simulink library "m_3SPS"  (R2017a)
settings: Solver=VariableStepAuto  StartTime=0.0  StopTime=10.0  RelTol=1e-3
libraries: mblibv1 x31
settings Model: Creator=ivanp7  LastModifiedBy=ivanp7

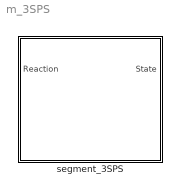
== system m_3SPS ==
  segment_3SPS : Subsystem  mask{segment_turn=0, platform_mass=0, platform_width=0, platform_thickness=0, platform_inertia=[0 0 0; 0 0 0; 0 0 0], mechanism_mass=0, mechanism_height=0, base_width=0, piston_mass=0, piston_inertia=[0 0 0; 0 0 0; 0 0 0], cylinder_inertia=[0 0 0; 0 0 0; 0 0 0]}
      mask prompts: segment_turn "Segment turn angle"; platform_mass "Platform mass, kg"; platform_width "Platform width, m"; platform_thickness "Platform thickness, m"; platform_inertia "Platform momentum of inertia matrix, kg*m^2"; mechanism_mass "Mechanism mass, kg"; mechanism_height "Mechanism height, m"; base_width "Base width, m"; piston_mass ""Piston" mass"; piston_inertia ""Piston" momentum of inertia matrix, kg*m^2"; cylinder_inertia ""Cylinder" momentum of inertia matrix, kg*m^2"
      mask init:
      | platform_radius = platform_width/2;
      | base_radius = base_width/2;
      | p_length = sqrt(mechanism_height^2 + (base_radius-platform_radius)^2);
      | 
      | q0 = [([1 1 1] * sign(base_radius-platform_radius) * sqrt((1 - mechanism_height / sqrt(mechanism_height^2 + (base_radius-platform_radius)^2)) / 2))  sqrt((1 + mechanism_height / sqrt(mechanism_height^2 + (base_radius-platform_radius)^2)) / 2)];
      | p1_quaternion = [[1 0 0] 1] .* q0;
      | p2_quaternion = [[-1/2 -sqrt(3)/2 0] 1] .* q0;
      | p3_quaternion = [[-1/2 sqrt(3)/2 0] 1] .* q0;
      | 
      | cylinder_mass = mechanism_mass/3 - piston_mass;
      mask DialogControl Container_plat_param Prompt: Platform parameters
      mask DialogControl Container_mech_param Prompt: Mechanism parameters
      mask DialogControl Container_mech_add_param Prompt: Additional mechanism parameters

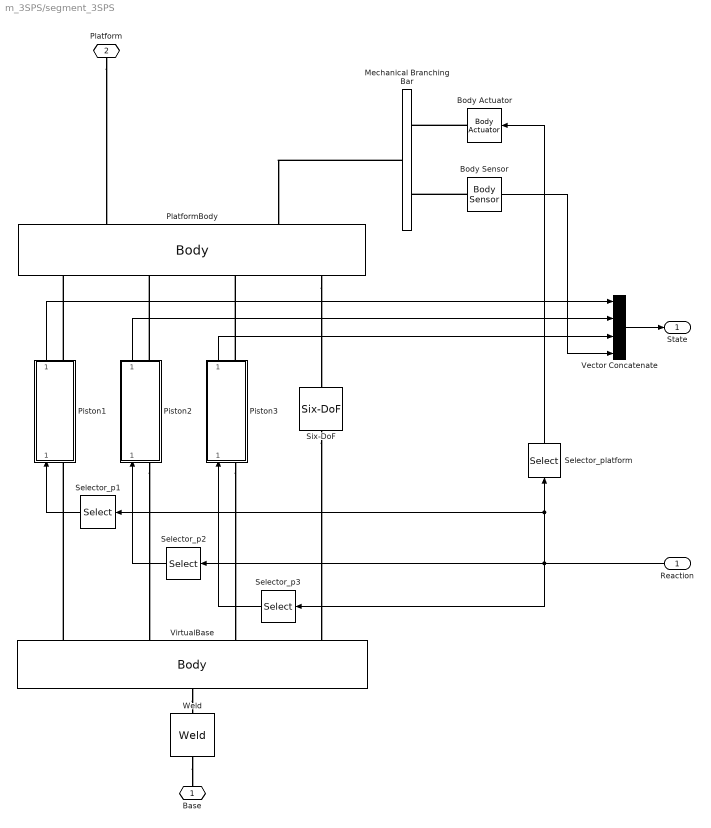
== system m_3SPS/segment_3SPS ==
  Reaction : Inport  OutDataTypeStr=double
  Body Actuator : mblibv1/Sensors &  Actuators/Body Actuator  UpdateFromCAD=off  PhysicalDomain=Mechanical  PortType=blob  ActuationStyle=Force  AngleUnits=deg  ArcVelocityUnits=deg/s  ArcAccelerationUnits=deg/s^2  CoordPositionUnits=m  VelocityUnits=m/s  AccelerationUnits=m/s^2  ForceUnits=N  TorqueUnits=N*m  ActiveIO=off  Width=1  DialogClass=MechanicalActuatorBlock  ReferenceFrame=Absolute (World)  Angle=off  CoordPosition=on  Force=on  Torque=on
      settings: SourceProductName=Simscape Multibody  SourceProductBaseCode=MS
  Body Sensor : mblibv1/Sensors &  Actuators/Body Sensor  UpdateFromCAD=off  PhysicalDomain=Mechanical  PortType=blob  Muxed=on  Pose=on  Angle=on  AngleUnits=deg  ArcVelocity=on  ArcVelocityUnits=rad/s  ArcAcceleration=on  ArcAccelerationUnits=rad/s^2  CoordPosition=on  CoordPositionUnits=m  Velocity=on  VelocityUnits=m/s  Acceleration=on  AccelerationUnits=m/s^2  Quaternion=on  QuaternionDT=off  QuaternionDDT=off  QuaternionUnits=off  OutputVector=[1]  ActiveIO=off  Width=1  DialogClass=MechanicalSensorBlock  ReferenceFrame=Absolute (World)
      settings: SourceProductName=Simscape Multibody  SourceProductBaseCode=MS
  Mechanical Branching Bar : mblibv1/Utilities/Mechanical Branching Bar  LConnTagsString=_newl0  RConnTagsString=SA0|SA1  UpdateFromCAD=off  DialogClass=MechanicalBranchingBarBlock  NumSAPorts=2
      settings: SourceProductName=Simscape Multibody  SourceProductBaseCode=MS
  Piston1 : Subsystem
  Piston2 : Subsystem
  Piston3 : Subsystem
  PlatformBody : mblibv1/Bodies/Body  LConnTagsString=CS5|CS6  RConnTagsString=CS1|CS2|CS3|CS4  UpdateFromCAD=off  DialogClass=MechanicalBodyBlock  Mass=platform_mass  MassUnits=kg  InertiaUnits=kg*m^2  Inertia=platform_inertia  Shape=Cylinder  ShapeDims=[1 1]  ShapeUnits=m  ShapeUse=false  Density=1  DensityUnits=kg/m^3  DensityUse=false  GraphicsMode=EQELLIPSE  BodyColorSelMode=MACHINE_DEFAULT  BodyColor=[1 0 0]  AttachedToCS=CG  CG=Left$CG$[0 0 platform_thickness/2]$CS4$CS4$m$[0 0 0]$Euler X-Y-Z$deg$CS4$false$none  WorkingFrames=Right$CS1$[0 0 0]$Adjoining$Adjoining$m$[0 0 0]$Euler X-Y-Z$deg$CS4$true$none#Right$CS2$[0 0 0]$Adjoining$Adjoining$m$[0 0 0]$Euler X-Y-Z$deg$CS4$true$none#Right$CS3$[0 0 0]$Adjoining$Adjoining$m$[0 0 0]$Euler X-Y-Z$deg$CS4$true$none#Right$CS4$[0 0 mechanism_height]$Adjoining$Adjoining$m$[0 0 0]$Euler X-Y-Z$deg$Adjoining$true$none#Left$CS5$[0 0 platform_thickness]$CS4$CS4$m$[0 0 0]$Euler X-Y-Z$deg$CS4$true$none#Left$CS6$[0 0 0]$CS5$CS5$m$[0 0 0]$Euler X-Y-Z$deg$CG$true$none  CGPos=[0 0 platform_thickness/2]  CGRot=[0 0 0]  CS0Pos=[]  CS0Rot=[]  CS1Pos=[0 0 0]  CS1Rot=[0 0 0]  CS2Pos=[0 0 0]  CS2Rot=[0 0 0]  CS3Pos=[0 0 0]  CS3Rot=[0 0 0]  CS4Pos=[0 0 mechanism_height]  CS4Rot=[0 0 0]  CS5Pos=[0 0 platform_thickness]  CS5Rot=[0 0 0]  CS6Pos=[0 0 0]  CS6Rot=[0 0 0]  CS7Pos=[]  CS7Rot=[]  CS8Pos=[]  CS8Rot=[]  CS9Pos=[]  CS9Rot=[]  CS10Pos=[]  CS10Rot=[]  CS11Pos=[]  CS11Rot=[]  CS12Pos=[]  CS12Rot=[]  CS13Pos=[]  CS13Rot=[]  CS14Pos=[]  CS14Rot=[]  CS15Pos=[]  CS15Rot=[]  CS16Pos=[]  CS16Rot=[]  CS17Pos=[]  CS17Rot=[]  CS18Pos=[]  CS18Rot=[]  CS19Pos=[]  CS19Rot=[]  CS20Pos=[]  CS20Rot=[]
      settings: SourceProductName=Simscape Multibody  SourceProductBaseCode=MS
  Selector_p1 : Selector  InputPortWidth=9  IndexOptions=Index vector (dialog)  Indices=[1]  OutputSizes=1
  Selector_p2 : Selector  InputPortWidth=9  IndexOptions=Index vector (dialog)  Indices=[2]  OutputSizes=1
  Selector_p3 : Selector  InputPortWidth=9  IndexOptions=Index vector (dialog)  Indices=[3]  OutputSizes=1
  Selector_platform : Selector  InputPortWidth=9  IndexOptions=Index vector (dialog)  Indices=[4 5 6 7 8 9]  OutputSizes=1
  Six-DoF : mblibv1/Joints/Six-DoF  LConnTagsString=__newl0  RConnTagsString=__newr0  UpdateFromCAD=off  NumSAPorts=0  CutJoint=off  MarkAsCut=off  Primitives=prismatic_prismatic  PrimitiveProps=P1$WORLD$[1 0 0]$prismatic#P2$WORLD$[0 1 0]$prismatic#P3$WORLD$[0 0 1]$prismatic#S$WORLD$[0 0 0]$spherical  DialogClass=JointBlock  P1Axis=[1 0 0]  P2Axis=[0 1 0]  P3Axis=[0 0 1]  SAxis=[0 0 0]
      settings: SourceProductName=Simscape Multibody  SourceProductBaseCode=MS
  Vector Concatenate : Concatenate  NumInputs=4
  VirtualBase : mblibv1/Bodies/Body  LConnTagsString=CS1|CS2|CS3|CS4  RConnTagsString=CG  UpdateFromCAD=off  DialogClass=MechanicalBodyBlock  Mass=0  MassUnits=kg  InertiaUnits=kg*m^2  Inertia=zeros(3)  Shape=Cylinder  ShapeDims=[1 1]  ShapeUnits=m  ShapeUse=false  Density=1  DensityUnits=kg/m^3  DensityUse=false  GraphicsMode=EQELLIPSE  BodyColorSelMode=MACHINE_DEFAULT  BodyColor=[1 0 0]  AttachedToCS=CG  CG=Right$CG$[0 0 0]$Adjoining$Adjoining$m$[0 0 segment_turn]$Euler X-Y-Z$deg$Adjoining$true$none  WorkingFrames=Left$CS1$[0 base_radius 0]$CG$CG$m$[0 0 0]$Euler X-Y-Z$deg$CG$true$none#Left$CS2$[sqrt(3)*base_radius/2 -base_radius/2 0]$CG$CG$m$[0 0 0]$Euler X-Y-Z$deg$CG$true$none#Left$CS3$[-sqrt(3)*base_radius/2 -base_radius/2 0]$CG$CG$m$[0 0 0]$Euler X-Y-Z$deg$CG$true$none#Left$CS4$[0 0 0]$CG$CG$m$[0 0 0]$Euler X-Y-Z$deg$CG$true$none  CGPos=[0 0 0]  CGRot=[0 0 segment_turn]  CS0Pos=[]  CS0Rot=[]  CS1Pos=[0 base_radius 0]  CS1Rot=[0 0 0]  CS2Pos=[sqrt(3)*base_radius/2 -base_radius/2 0]  CS2Rot=[0 0 0]  CS3Pos=[-sqrt(3)*base_radius/2 -base_radius/2 0]  CS3Rot=[0 0 0]  CS4Pos=[0 0 0]  CS4Rot=[0 0 0]  CS5Pos=[]  CS5Rot=[]  CS6Pos=[]  CS6Rot=[]  CS7Pos=[]  CS7Rot=[]  CS8Pos=[]  CS8Rot=[]  CS9Pos=[]  CS9Rot=[]  CS10Pos=[]  CS10Rot=[]  CS11Pos=[]  CS11Rot=[]  CS12Pos=[]  CS12Rot=[]  CS13Pos=[]  CS13Rot=[]  CS14Pos=[]  CS14Rot=[]  CS15Pos=[]  CS15Rot=[]  CS16Pos=[]  CS16Rot=[]  CS17Pos=[]  CS17Rot=[]  CS18Pos=[]  CS18Rot=[]  CS19Pos=[]  CS19Rot=[]  CS20Pos=[]  CS20Rot=[]
      settings: SourceProductName=Simscape Multibody  SourceProductBaseCode=MS
  Weld : mblibv1/Joints/Weld  LConnTagsString=__newl0  RConnTagsString=__newr0  UpdateFromCAD=off  NumSAPorts=0  CutJoint=off  MarkAsCut=off  Primitives=weld  PrimitiveProps=W$WORLD$[0 0 0]$weld  DialogClass=JointBlock  WAxis=[0 0 0]
      settings: SourceProductName=Simscape Multibody  SourceProductBaseCode=MS
  Base : PMIOPort  Port=1  Side=Left
  Platform : PMIOPort  Port=2  Side=Right
  State : Outport  OutDataTypeStr=double
  wires:
  Piston1/1(P1_State) -> Vector Concatenate/1
  Piston2/1(P2_State) -> Vector Concatenate/2
  Piston3/1(P3_State) -> Vector Concatenate/3
  Reaction/1 -> Selector_p3/1, Selector_p1/1, Selector_platform/1, Selector_p2/1
  Vector Concatenate/1 -> State/1
  Body Sensor/1 -> Vector Concatenate/4
  Selector_platform/1 -> Body Actuator/1
  Selector_p1/1 -> Piston1/1(P1_Reaction)
  Selector_p2/1 -> Piston2/1(P2_Reaction)
  Selector_p3/1 -> Piston3/1(P3_Reaction)
  connections:
  Weld/LConn1 -- Base/RConn1
  VirtualBase/RConn1 -- Weld/RConn1
  Piston1/RConn1 -- PlatformBody/RConn1
  VirtualBase/LConn1 -- Piston1/LConn1
  Six-DoF/LConn1 -- VirtualBase/LConn4
  Platform/RConn1 -- PlatformBody/LConn1
  PlatformBody/RConn4 -- Six-DoF/RConn1
  Piston2/LConn1 -- VirtualBase/LConn2
  Piston2/RConn1 -- PlatformBody/RConn2
  Piston3/RConn1 -- PlatformBody/RConn3
  Piston3/LConn1 -- VirtualBase/LConn3
  Body Actuator/RConn1 -- Mechanical Branching Bar/RConn1
  Body Sensor/LConn1 -- Mechanical Branching Bar/RConn2
  Mechanical Branching Bar/LConn1 -- PlatformBody/LConn2

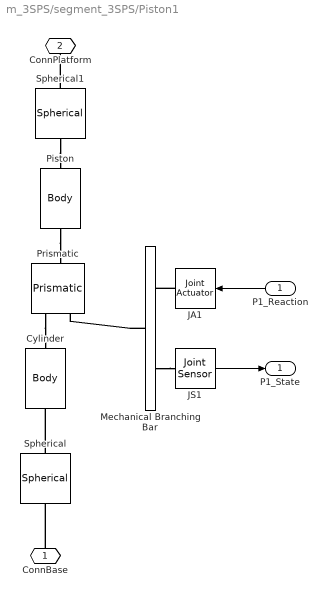
== system m_3SPS/segment_3SPS/Piston1 ==
  P1_Reaction : Inport
  Cylinder : mblibv1/Bodies/Body  LConnTagsString=CG  RConnTagsString=CS2  UpdateFromCAD=off  DialogClass=MechanicalBodyBlock  Mass=cylinder_mass  MassUnits=kg  InertiaUnits=kg*m^2  Inertia=cylinder_inertia  Shape=Cylinder  ShapeDims=[1 1]  ShapeUnits=m  ShapeUse=false  Density=1  DensityUnits=kg/m^3  DensityUse=false  GraphicsMode=MACHINE_DEFAULT  BodyColorSelMode=MACHINE_DEFAULT  BodyColor=[1 0 0]  AttachedToCS=CG  CG=Left$CG$[0 0 p_length/2]$CS2$CS2$m$[0 0 0]$Euler X-Y-Z$deg$CS2$true$none  WorkingFrames=Left$CS1$[0 0 p_length]$CS2$CS2$m$[0 0 0]$Euler X-Y-Z$deg$CS2$false$none#Right$CS2$[0 0 0]$Adjoining$Adjoining$m$p1_quaternion$Quaternion$rad$Adjoining$true$none  CGPos=[0 0 p_length/2]  CGRot=[0 0 0]  CS0Pos=[]  CS0Rot=[]  CS1Pos=[0 0 p_length]  CS1Rot=[0 0 0]  CS2Pos=[0 0 0]  CS2Rot=p1_quaternion  CS3Pos=[]  CS3Rot=[]  CS4Pos=[]  CS4Rot=[]  CS5Pos=[]  CS5Rot=[]  CS6Pos=[]  CS6Rot=[]  CS7Pos=[]  CS7Rot=[]  CS8Pos=[]  CS8Rot=[]  CS9Pos=[]  CS9Rot=[]  CS10Pos=[]  CS10Rot=[]  CS11Pos=[]  CS11Rot=[]  CS12Pos=[]  CS12Rot=[]  CS13Pos=[]  CS13Rot=[]  CS14Pos=[]  CS14Rot=[]  CS15Pos=[]  CS15Rot=[]  CS16Pos=[]  CS16Rot=[]  CS17Pos=[]  CS17Rot=[]  CS18Pos=[]  CS18Rot=[]  CS19Pos=[]  CS19Rot=[]  CS20Pos=[]  CS20Rot=[]
      settings: SourceProductName=Simscape Multibody  SourceProductBaseCode=MS
  JA1 : mblibv1/Sensors &  Actuators/Joint Actuator  UpdateFromCAD=off  PhysicalDomain=Mechanical  PortType=blob  ActuationStyle=Force  AngleUnits=rad  ArcVelocityUnits=rad/s  ArcAccelerationUnits=rad/s^2  CoordPositionUnits=cm  VelocityUnits=m/s  AccelerationUnits=m/s^2  ForceUnits=N  TorqueUnits=N*m  ActiveIO=off  Width=1  DialogClass=MechanicalActuatorBlock  Primitive=P1  ReferenceFrame=Absolute (World)
      settings: SourceProductName=Simscape Multibody  SourceProductBaseCode=MS
  JS1 : mblibv1/Sensors &  Actuators/Joint Sensor  UpdateFromCAD=off  PhysicalDomain=Mechanical  PortType=blob  Muxed=on  Pose=off  Angle=on  AngleUnits=rad  ArcVelocity=on  ArcVelocityUnits=rad/s  ArcAcceleration=on  ArcAccelerationUnits=rad/s^2  CoordPosition=on  CoordPositionUnits=m  Velocity=on  VelocityUnits=m/s  Acceleration=on  AccelerationUnits=m/s^2  Quaternion=on  QuaternionDT=off  QuaternionDDT=off  QuaternionUnits=off  OutputVector=[1]  ActiveIO=off  Width=1  DialogClass=MechanicalSensorBlock  Primitive=P1  Force=on  ForceUnits=N  Torque=on  TorqueUnits=N*m  ReferenceFrame=Absolute (World)  ReactionSensedSide=Base  ReactionReferenceFrame=Local (Body CS)  ReactionForce=on  ReactionForceUnits=N  ReactionMoment=on  ReactionMomentUnits=N*m
      settings: SourceProductName=Simscape Multibody  SourceProductBaseCode=MS
  Mechanical Branching Bar : mblibv1/Utilities/Mechanical Branching Bar  LConnTagsString=_newl0  RConnTagsString=SA0|SA1  UpdateFromCAD=off  DialogClass=MechanicalBranchingBarBlock  NumSAPorts=2
      settings: SourceProductName=Simscape Multibody  SourceProductBaseCode=MS
  Piston : mblibv1/Bodies/Body  LConnTagsString=CS1  RConnTagsString=CG  UpdateFromCAD=off  DialogClass=MechanicalBodyBlock  Mass=piston_mass  MassUnits=kg  InertiaUnits=kg*m^2  Inertia=piston_inertia  Shape=Cylinder  ShapeDims=[1 1]  ShapeUnits=m  ShapeUse=false  Density=1  DensityUnits=kg/m^3  DensityUse=false  GraphicsMode=MACHINE_DEFAULT  BodyColorSelMode=MACHINE_DEFAULT  BodyColor=[1 0 0]  AttachedToCS=CG  CG=Right$CG$[0 0 0]$Adjoining$Adjoining$m$[0 0 0]$Euler X-Y-Z$deg$Adjoining$true$none  WorkingFrames=Left$CS1$[0 0 p_length/2]$CG$CG$m$[0 0 0]$Euler X-Y-Z$deg$CG$true$none#Right$CS2$[0 0 -p_length/2]$CG$CG$m$[0 0 0]$Euler X-Y-Z$deg$CG$false$none  CGPos=[0 0 0]  CGRot=[0 0 0]  CS0Pos=[]  CS0Rot=[]  CS1Pos=[0 0 p_length/2]  CS1Rot=[0 0 0]  CS2Pos=[0 0 -p_length/2]  CS2Rot=[0 0 0]  CS3Pos=[]  CS3Rot=[]  CS4Pos=[]  CS4Rot=[]  CS5Pos=[]  CS5Rot=[]  CS6Pos=[]  CS6Rot=[]  CS7Pos=[]  CS7Rot=[]  CS8Pos=[]  CS8Rot=[]  CS9Pos=[]  CS9Rot=[]  CS10Pos=[]  CS10Rot=[]  CS11Pos=[]  CS11Rot=[]  CS12Pos=[]  CS12Rot=[]  CS13Pos=[]  CS13Rot=[]  CS14Pos=[]  CS14Rot=[]  CS15Pos=[]  CS15Rot=[]  CS16Pos=[]  CS16Rot=[]  CS17Pos=[]  CS17Rot=[]  CS18Pos=[]  CS18Rot=[]  CS19Pos=[]  CS19Rot=[]  CS20Pos=[]  CS20Rot=[]
      settings: SourceProductName=Simscape Multibody  SourceProductBaseCode=MS
  Prismatic : mblibv1/Joints/Prismatic  LConnTagsString=__newl0|SA1  RConnTagsString=__newr0  UpdateFromCAD=off  NumSAPorts=1  CutJoint=off  MarkAsCut=off  Primitives=prismatic  PrimitiveProps=P1$Base$[0 0 1]$prismatic  DialogClass=JointBlock  P1Axis=[0 0 1]
      settings: SourceProductName=Simscape Multibody  SourceProductBaseCode=MS
  Spherical : mblibv1/Joints/Spherical  LConnTagsString=__newl0  RConnTagsString=__newr0  UpdateFromCAD=off  NumSAPorts=0  CutJoint=off  MarkAsCut=off  Primitives=spherical  PrimitiveProps=S$WORLD$[0 0 0]$spherical  DialogClass=JointBlock  SAxis=[0 0 0]
      settings: SourceProductName=Simscape Multibody  SourceProductBaseCode=MS
  Spherical1 : mblibv1/Joints/Spherical  LConnTagsString=__newl0  RConnTagsString=__newr0  UpdateFromCAD=off  NumSAPorts=0  CutJoint=off  MarkAsCut=off  Primitives=spherical  PrimitiveProps=S$WORLD$[0 0 0]$spherical  DialogClass=JointBlock  SAxis=[0 0 0]
      settings: SourceProductName=Simscape Multibody  SourceProductBaseCode=MS
  ConnBase : PMIOPort  Port=1  Side=Left
  ConnPlatform : PMIOPort  Port=2  Side=Right
  P1_State : Outport
  wires:
  JS1/1 -> P1_State/1
  P1_Reaction/1 -> JA1/1
  connections:
  ConnBase/RConn1 -- Spherical/LConn1
  Piston/RConn1 -- Prismatic/RConn1
  Spherical1/RConn1 -- ConnPlatform/RConn1
  Prismatic/LConn1 -- Cylinder/LConn1
  Spherical1/LConn1 -- Piston/LConn1
  Spherical/RConn1 -- Cylinder/RConn1
  Mechanical Branching Bar/RConn2 -- JS1/LConn1
  JA1/RConn1 -- Mechanical Branching Bar/RConn1
  Mechanical Branching Bar/LConn1 -- Prismatic/LConn2

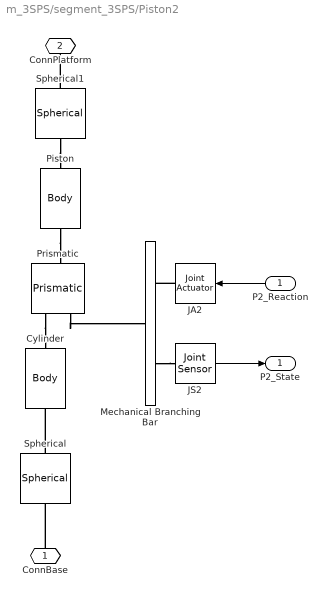
== system m_3SPS/segment_3SPS/Piston2 ==
  P2_Reaction : Inport
  Cylinder : mblibv1/Bodies/Body  LConnTagsString=CG  RConnTagsString=CS2  UpdateFromCAD=off  DialogClass=MechanicalBodyBlock  Mass=cylinder_mass  MassUnits=kg  InertiaUnits=kg*m^2  Inertia=cylinder_inertia  Shape=Cylinder  ShapeDims=[1 1]  ShapeUnits=m  ShapeUse=false  Density=1  DensityUnits=kg/m^3  DensityUse=false  GraphicsMode=MACHINE_DEFAULT  BodyColorSelMode=MACHINE_DEFAULT  BodyColor=[1 0 0]  AttachedToCS=CG  CG=Left$CG$[0 0 p_length/2]$CS2$CS2$m$[0 0 0]$Euler X-Y-Z$deg$CS2$true$none  WorkingFrames=Left$CS1$[0 0 p_length]$CS2$CS2$m$[0 0 0]$Euler X-Y-Z$deg$CS2$false$none#Right$CS2$[0 0 0]$Adjoining$Adjoining$m$p2_quaternion$Quaternion$rad$Adjoining$true$none  CGPos=[0 0 p_length/2]  CGRot=[0 0 0]  CS0Pos=[]  CS0Rot=[]  CS1Pos=[0 0 p_length]  CS1Rot=[0 0 0]  CS2Pos=[0 0 0]  CS2Rot=p2_quaternion  CS3Pos=[]  CS3Rot=[]  CS4Pos=[]  CS4Rot=[]  CS5Pos=[]  CS5Rot=[]  CS6Pos=[]  CS6Rot=[]  CS7Pos=[]  CS7Rot=[]  CS8Pos=[]  CS8Rot=[]  CS9Pos=[]  CS9Rot=[]  CS10Pos=[]  CS10Rot=[]  CS11Pos=[]  CS11Rot=[]  CS12Pos=[]  CS12Rot=[]  CS13Pos=[]  CS13Rot=[]  CS14Pos=[]  CS14Rot=[]  CS15Pos=[]  CS15Rot=[]  CS16Pos=[]  CS16Rot=[]  CS17Pos=[]  CS17Rot=[]  CS18Pos=[]  CS18Rot=[]  CS19Pos=[]  CS19Rot=[]  CS20Pos=[]  CS20Rot=[]
      settings: SourceProductName=Simscape Multibody  SourceProductBaseCode=MS
  JA2 : mblibv1/Sensors &  Actuators/Joint Actuator  UpdateFromCAD=off  PhysicalDomain=Mechanical  PortType=blob  ActuationStyle=Force  AngleUnits=rad  ArcVelocityUnits=rad/s  ArcAccelerationUnits=rad/s^2  CoordPositionUnits=mm  VelocityUnits=m/s  AccelerationUnits=m/s^2  ForceUnits=N  TorqueUnits=N*m  ActiveIO=off  Width=1  DialogClass=MechanicalActuatorBlock  Primitive=P1  ReferenceFrame=Absolute (World)
      settings: SourceProductName=Simscape Multibody  SourceProductBaseCode=MS
  JS2 : mblibv1/Sensors &  Actuators/Joint Sensor  UpdateFromCAD=off  PhysicalDomain=Mechanical  PortType=blob  Muxed=on  Pose=off  Angle=on  AngleUnits=rad  ArcVelocity=on  ArcVelocityUnits=rad/s  ArcAcceleration=on  ArcAccelerationUnits=rad/s^2  CoordPosition=on  CoordPositionUnits=m  Velocity=on  VelocityUnits=m/s  Acceleration=on  AccelerationUnits=m/s^2  Quaternion=on  QuaternionDT=off  QuaternionDDT=off  QuaternionUnits=off  OutputVector=[1]  ActiveIO=off  Width=1  DialogClass=MechanicalSensorBlock  Primitive=P1  Force=on  ForceUnits=N  Torque=on  TorqueUnits=N*m  ReferenceFrame=Absolute (World)  ReactionSensedSide=Base  ReactionReferenceFrame=Local (Body CS)  ReactionForce=on  ReactionForceUnits=N  ReactionMoment=on  ReactionMomentUnits=N*m
      settings: SourceProductName=Simscape Multibody  SourceProductBaseCode=MS
  Mechanical Branching Bar : mblibv1/Utilities/Mechanical Branching Bar  LConnTagsString=_newl0  RConnTagsString=SA0|SA1  UpdateFromCAD=off  DialogClass=MechanicalBranchingBarBlock  NumSAPorts=2
      settings: SourceProductName=Simscape Multibody  SourceProductBaseCode=MS
  Piston : mblibv1/Bodies/Body  LConnTagsString=CS1  RConnTagsString=CG  UpdateFromCAD=off  DialogClass=MechanicalBodyBlock  Mass=piston_mass  MassUnits=kg  InertiaUnits=kg*m^2  Inertia=piston_inertia  Shape=Cylinder  ShapeDims=[1 1]  ShapeUnits=m  ShapeUse=false  Density=1  DensityUnits=kg/m^3  DensityUse=false  GraphicsMode=MACHINE_DEFAULT  BodyColorSelMode=MACHINE_DEFAULT  BodyColor=[1 0 0]  AttachedToCS=CG  CG=Right$CG$[0 0 0]$Adjoining$Adjoining$m$[0 0 0]$Euler X-Y-Z$deg$Adjoining$true$none  WorkingFrames=Left$CS1$[0 0 p_length/2]$CG$CG$m$[0 0 0]$Euler X-Y-Z$deg$CG$true$none#Right$CS2$[0 0 -p_length/2]$CG$CG$m$[0 0 0]$Euler X-Y-Z$deg$CG$false$none  CGPos=[0 0 0]  CGRot=[0 0 0]  CS0Pos=[]  CS0Rot=[]  CS1Pos=[0 0 p_length/2]  CS1Rot=[0 0 0]  CS2Pos=[0 0 -p_length/2]  CS2Rot=[0 0 0]  CS3Pos=[]  CS3Rot=[]  CS4Pos=[]  CS4Rot=[]  CS5Pos=[]  CS5Rot=[]  CS6Pos=[]  CS6Rot=[]  CS7Pos=[]  CS7Rot=[]  CS8Pos=[]  CS8Rot=[]  CS9Pos=[]  CS9Rot=[]  CS10Pos=[]  CS10Rot=[]  CS11Pos=[]  CS11Rot=[]  CS12Pos=[]  CS12Rot=[]  CS13Pos=[]  CS13Rot=[]  CS14Pos=[]  CS14Rot=[]  CS15Pos=[]  CS15Rot=[]  CS16Pos=[]  CS16Rot=[]  CS17Pos=[]  CS17Rot=[]  CS18Pos=[]  CS18Rot=[]  CS19Pos=[]  CS19Rot=[]  CS20Pos=[]  CS20Rot=[]
      settings: SourceProductName=Simscape Multibody  SourceProductBaseCode=MS
  Prismatic : mblibv1/Joints/Prismatic  LConnTagsString=__newl0|SA1  RConnTagsString=__newr0  UpdateFromCAD=off  NumSAPorts=1  CutJoint=off  MarkAsCut=off  Primitives=prismatic  PrimitiveProps=P1$Base$[0 0 1]$prismatic  DialogClass=JointBlock  P1Axis=[0 0 1]
      settings: SourceProductName=Simscape Multibody  SourceProductBaseCode=MS
  Spherical : mblibv1/Joints/Spherical  LConnTagsString=__newl0  RConnTagsString=__newr0  UpdateFromCAD=off  NumSAPorts=0  CutJoint=off  MarkAsCut=off  Primitives=spherical  PrimitiveProps=S$WORLD$[0 0 0]$spherical  DialogClass=JointBlock  SAxis=[0 0 0]
      settings: SourceProductName=Simscape Multibody  SourceProductBaseCode=MS
  Spherical1 : mblibv1/Joints/Spherical  LConnTagsString=__newl0  RConnTagsString=__newr0  UpdateFromCAD=off  NumSAPorts=0  CutJoint=off  MarkAsCut=off  Primitives=spherical  PrimitiveProps=S$WORLD$[0 0 0]$spherical  DialogClass=JointBlock  SAxis=[0 0 0]
      settings: SourceProductName=Simscape Multibody  SourceProductBaseCode=MS
  ConnBase : PMIOPort  Port=1  Side=Left
  ConnPlatform : PMIOPort  Port=2  Side=Right
  P2_State : Outport
  wires:
  P2_Reaction/1 -> JA2/1
  JS2/1 -> P2_State/1
  connections:
  Spherical/RConn1 -- Cylinder/RConn1
  Spherical1/LConn1 -- Piston/LConn1
  Prismatic/LConn1 -- Cylinder/LConn1
  Spherical1/RConn1 -- ConnPlatform/RConn1
  Piston/RConn1 -- Prismatic/RConn1
  ConnBase/RConn1 -- Spherical/LConn1
  Mechanical Branching Bar/RConn2 -- JS2/LConn1
  JA2/RConn1 -- Mechanical Branching Bar/RConn1
  Prismatic/LConn2 -- Mechanical Branching Bar/LConn1

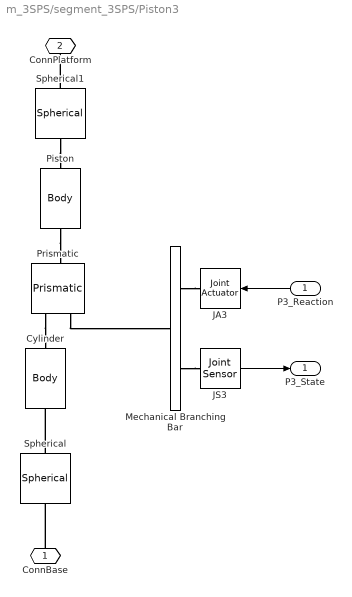
== system m_3SPS/segment_3SPS/Piston3 ==
  P3_Reaction : Inport
  Cylinder : mblibv1/Bodies/Body  LConnTagsString=CG  RConnTagsString=CS2  UpdateFromCAD=off  DialogClass=MechanicalBodyBlock  Mass=cylinder_mass  MassUnits=kg  InertiaUnits=kg*m^2  Inertia=cylinder_inertia  Shape=Cylinder  ShapeDims=[1 1]  ShapeUnits=m  ShapeUse=false  Density=1  DensityUnits=kg/m^3  DensityUse=false  GraphicsMode=MACHINE_DEFAULT  BodyColorSelMode=MACHINE_DEFAULT  BodyColor=[1 0 0]  AttachedToCS=CG  CG=Left$CG$[0 0 p_length/2]$CS2$CS2$m$[0 0 0]$Euler X-Y-Z$deg$CS2$true$none  WorkingFrames=Left$CS1$[0 0 p_length]$CS2$CS2$m$[0 0 0]$Euler X-Y-Z$deg$CS2$false$none#Right$CS2$[0 0 0]$Adjoining$Adjoining$m$p3_quaternion$Quaternion$rad$Adjoining$true$none  CGPos=[0 0 p_length/2]  CGRot=[0 0 0]  CS0Pos=[]  CS0Rot=[]  CS1Pos=[0 0 p_length]  CS1Rot=[0 0 0]  CS2Pos=[0 0 0]  CS2Rot=p3_quaternion  CS3Pos=[]  CS3Rot=[]  CS4Pos=[]  CS4Rot=[]  CS5Pos=[]  CS5Rot=[]  CS6Pos=[]  CS6Rot=[]  CS7Pos=[]  CS7Rot=[]  CS8Pos=[]  CS8Rot=[]  CS9Pos=[]  CS9Rot=[]  CS10Pos=[]  CS10Rot=[]  CS11Pos=[]  CS11Rot=[]  CS12Pos=[]  CS12Rot=[]  CS13Pos=[]  CS13Rot=[]  CS14Pos=[]  CS14Rot=[]  CS15Pos=[]  CS15Rot=[]  CS16Pos=[]  CS16Rot=[]  CS17Pos=[]  CS17Rot=[]  CS18Pos=[]  CS18Rot=[]  CS19Pos=[]  CS19Rot=[]  CS20Pos=[]  CS20Rot=[]
      settings: SourceProductName=Simscape Multibody  SourceProductBaseCode=MS
  JA3 : mblibv1/Sensors &  Actuators/Joint Actuator  UpdateFromCAD=off  PhysicalDomain=Mechanical  PortType=blob  ActuationStyle=Force  AngleUnits=rad  ArcVelocityUnits=rad/s  ArcAccelerationUnits=rad/s^2  CoordPositionUnits=cm  VelocityUnits=m/s  AccelerationUnits=m/s^2  ForceUnits=N  TorqueUnits=N*m  ActiveIO=off  Width=1  DialogClass=MechanicalActuatorBlock  Primitive=P1  ReferenceFrame=Absolute (World)
      settings: SourceProductName=Simscape Multibody  SourceProductBaseCode=MS
  JS3 : mblibv1/Sensors &  Actuators/Joint Sensor  UpdateFromCAD=off  PhysicalDomain=Mechanical  PortType=blob  Muxed=on  Pose=off  Angle=on  AngleUnits=rad  ArcVelocity=on  ArcVelocityUnits=rad/s  ArcAcceleration=on  ArcAccelerationUnits=rad/s^2  CoordPosition=on  CoordPositionUnits=m  Velocity=on  VelocityUnits=m/s  Acceleration=on  AccelerationUnits=m/s^2  Quaternion=on  QuaternionDT=off  QuaternionDDT=off  QuaternionUnits=off  OutputVector=[1]  ActiveIO=off  Width=1  DialogClass=MechanicalSensorBlock  Primitive=P1  Force=on  ForceUnits=N  Torque=on  TorqueUnits=N*m  ReferenceFrame=Absolute (World)  ReactionSensedSide=Base  ReactionReferenceFrame=Local (Body CS)  ReactionForce=on  ReactionForceUnits=N  ReactionMoment=on  ReactionMomentUnits=N*m
      settings: SourceProductName=Simscape Multibody  SourceProductBaseCode=MS
  Mechanical Branching Bar : mblibv1/Utilities/Mechanical Branching Bar  LConnTagsString=_newl0  RConnTagsString=SA0|SA1  UpdateFromCAD=off  DialogClass=MechanicalBranchingBarBlock  NumSAPorts=2
      settings: SourceProductName=Simscape Multibody  SourceProductBaseCode=MS
  Piston : mblibv1/Bodies/Body  LConnTagsString=CS1  RConnTagsString=CG  UpdateFromCAD=off  DialogClass=MechanicalBodyBlock  Mass=piston_mass  MassUnits=kg  InertiaUnits=kg*m^2  Inertia=piston_inertia  Shape=Cylinder  ShapeDims=[1 1]  ShapeUnits=m  ShapeUse=false  Density=1  DensityUnits=kg/m^3  DensityUse=false  GraphicsMode=MACHINE_DEFAULT  BodyColorSelMode=MACHINE_DEFAULT  BodyColor=[1 0 0]  AttachedToCS=CG  CG=Right$CG$[0 0 0]$Adjoining$Adjoining$m$[0 0 0]$Euler X-Y-Z$deg$Adjoining$true$none  WorkingFrames=Left$CS1$[0 0 p_length/2]$CG$CG$m$[0 0 0]$Euler X-Y-Z$deg$CG$true$none#Right$CS2$[0 0 -p_length/2]$CG$CG$m$[0 0 0]$Euler X-Y-Z$deg$CG$false$none  CGPos=[0 0 0]  CGRot=[0 0 0]  CS0Pos=[]  CS0Rot=[]  CS1Pos=[0 0 p_length/2]  CS1Rot=[0 0 0]  CS2Pos=[0 0 -p_length/2]  CS2Rot=[0 0 0]  CS3Pos=[]  CS3Rot=[]  CS4Pos=[]  CS4Rot=[]  CS5Pos=[]  CS5Rot=[]  CS6Pos=[]  CS6Rot=[]  CS7Pos=[]  CS7Rot=[]  CS8Pos=[]  CS8Rot=[]  CS9Pos=[]  CS9Rot=[]  CS10Pos=[]  CS10Rot=[]  CS11Pos=[]  CS11Rot=[]  CS12Pos=[]  CS12Rot=[]  CS13Pos=[]  CS13Rot=[]  CS14Pos=[]  CS14Rot=[]  CS15Pos=[]  CS15Rot=[]  CS16Pos=[]  CS16Rot=[]  CS17Pos=[]  CS17Rot=[]  CS18Pos=[]  CS18Rot=[]  CS19Pos=[]  CS19Rot=[]  CS20Pos=[]  CS20Rot=[]
      settings: SourceProductName=Simscape Multibody  SourceProductBaseCode=MS
  Prismatic : mblibv1/Joints/Prismatic  LConnTagsString=__newl0|SA1  RConnTagsString=__newr0  UpdateFromCAD=off  NumSAPorts=1  CutJoint=off  MarkAsCut=off  Primitives=prismatic  PrimitiveProps=P1$Base$[0 0 1]$prismatic  DialogClass=JointBlock  P1Axis=[0 0 1]
      settings: SourceProductName=Simscape Multibody  SourceProductBaseCode=MS
  Spherical : mblibv1/Joints/Spherical  LConnTagsString=__newl0  RConnTagsString=__newr0  UpdateFromCAD=off  NumSAPorts=0  CutJoint=off  MarkAsCut=off  Primitives=spherical  PrimitiveProps=S$WORLD$[0 0 0]$spherical  DialogClass=JointBlock  SAxis=[0 0 0]
      settings: SourceProductName=Simscape Multibody  SourceProductBaseCode=MS
  Spherical1 : mblibv1/Joints/Spherical  LConnTagsString=__newl0  RConnTagsString=__newr0  UpdateFromCAD=off  NumSAPorts=0  CutJoint=off  MarkAsCut=off  Primitives=spherical  PrimitiveProps=S$WORLD$[0 0 0]$spherical  DialogClass=JointBlock  SAxis=[0 0 0]
      settings: SourceProductName=Simscape Multibody  SourceProductBaseCode=MS
  ConnBase : PMIOPort  Port=1  Side=Left
  ConnPlatform : PMIOPort  Port=2  Side=Right
  P3_State : Outport
  wires:
  JS3/1 -> P3_State/1
  P3_Reaction/1 -> JA3/1
  connections:
  ConnBase/RConn1 -- Spherical/LConn1
  Piston/RConn1 -- Prismatic/RConn1
  Spherical1/RConn1 -- ConnPlatform/RConn1
  Prismatic/LConn1 -- Cylinder/LConn1
  Spherical1/LConn1 -- Piston/LConn1
  Spherical/RConn1 -- Cylinder/RConn1
  Mechanical Branching Bar/RConn1 -- JA3/RConn1
  Mechanical Branching Bar/RConn2 -- JS3/LConn1
  Prismatic/LConn2 -- Mechanical Branching Bar/LConn1
